simulink subsystem "Day2_Scenario_2_3"  (R2024a)
settings: Solver=VariableStepAuto  StartTime=0.0  StopTime=10.0  RelTol=1e-3
libraries: CarMaker4SL x5
settings Model: Creator=junhyung.cha  LastModifiedBy=User

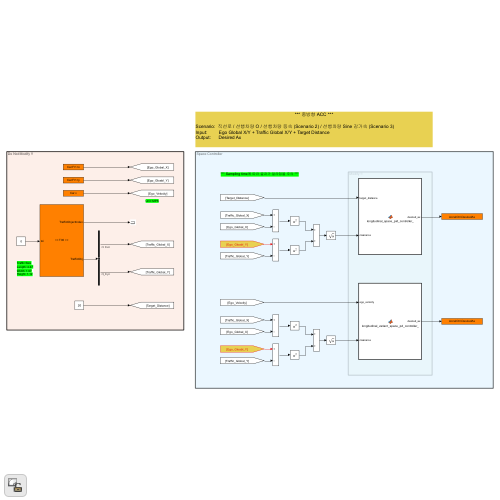
[thumbnail: Simulink's stored preview of the top-level diagram]
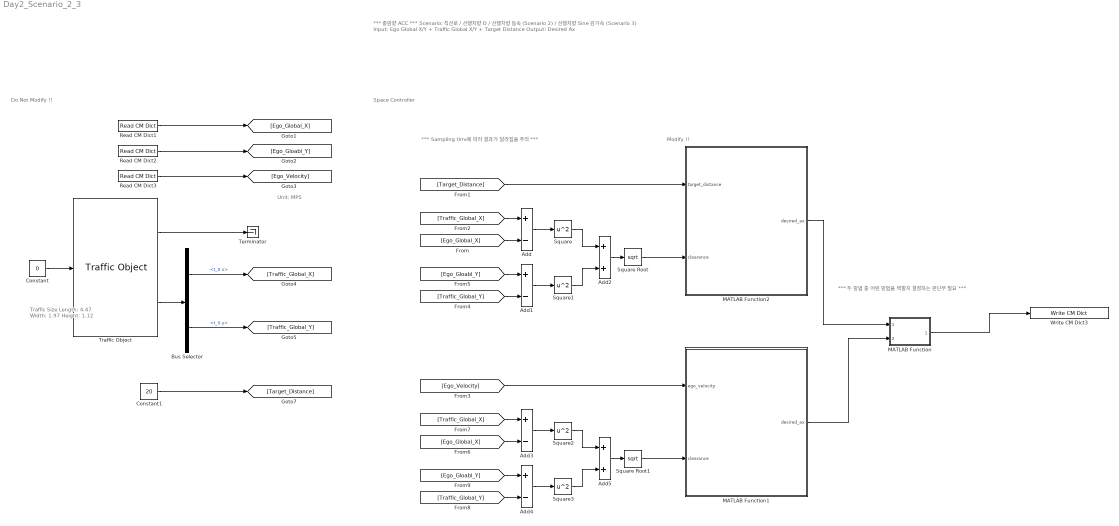
== system Day2_Scenario_2_3 ==
  note: *** Sampling time에 따라 결과가 달라짐을 주의 ***
  note: Space Controller
  note: Modify !!
  note: Do Not Modify !!
  note: Traffic Size
      | Length: 4.47
      | Width: 1.97
      | Height: 1.12
  note: *** 종방향 ACC ***
      |
      | Scenario: 직선로 / 선행차량 O / 선행차량 등속 (Scenario 2) / 선행차량 Sine 감가속 (Scenario 3)
      | Input: Ego Global X/Y + Traffic Global X/Y + Target Distance
      | Output: Desired Ax
  note: Unit: MPS
  note: *** 두 방법 중 어떤 방법을 택할지 결정하는 판단부 필요 ***
  Add{,1,3..4} (4 alike) : Sum  Inputs=+-
  Add2 : Sum
  Add5 : Sum
  Bus Selector : BusSelector  OutputSignals=t_0 x,t_0 y
  Constant : Constant  Value=0
  Constant1 : Constant  Value=20
  MATLAB Function : MATLAB Function  TreatAsAtomicUnit=on
  MATLAB Function1 : MATLAB Function  TreatAsAtomicUnit=on
  MATLAB Function2 : MATLAB Function  TreatAsAtomicUnit=on
  Read CM Dict1 : CarMaker4SL/Read CM Dict  xname=Car.Fr1.tx  xsync=off  xstime=Inherited
  Read CM Dict2 : CarMaker4SL/Read CM Dict  xname=Car.Fr1.ty  xsync=off  xstime=Inherited
  Read CM Dict3 : CarMaker4SL/Read CM Dict  xname=Car.v  xsync=off  xstime=Inherited
  Square{,1..3} (4 alike) : Math  Operator=square
  Square Root : Sqrt
  Square Root1 : Sqrt
  Terminator : Terminator
  Traffic Object : CarMaker4SL/Traffic Object  xname=T00  ximode=Traffic Id  xstime=Inherited
      settings: SourceProductName=CarMaker4SL
  Write CM Dict3 : CarMaker4SL/Write CM Dict  xname=AccelCtrl.DesiredAx  xsync=off
  wires:
  Read CM Dict2/1 -> [Ego_Gloabl_Y]
  Read CM Dict1/1 -> [Ego_Global_X]
  Constant/1 -> Traffic Object/1
  Traffic Object/2 -> Bus Selector/1
  Traffic Object/1 -> Terminator/1
  Bus Selector/1 -> [Traffic_Global_X]  "<t_0 x>"
  Bus Selector/2 -> [Traffic_Global_Y]  "<t_0 y>"
  Square Root/1 -> MATLAB Function2/2(clearance)
  Constant1/1 -> [Target_Distance]
  [Ego_Global_X] -> Add/2
  [Traffic_Global_X] -> Add/1
  [Traffic_Global_Y] -> Add1/2
  [Ego_Gloabl_Y] -> Add1/1
  Add1/1 -> Square1/1
  Add2/1 -> Square Root/1
  Square/1 -> Add2/1
  Square1/1 -> Add2/2
  [Target_Distance] -> MATLAB Function2/1(target_distance)
  Add/1 -> Square/1
  Read CM Dict3/1 -> [Ego_Velocity]
  [Ego_Velocity] -> MATLAB Function1/1(ego_velocity)
  Add3/1 -> Square2/1
  Square3/1 -> Add5/2
  Square2/1 -> Add5/1
  Add5/1 -> Square Root1/1
  Add4/1 -> Square3/1
  [Ego_Gloabl_Y] -> Add4/1
  [Traffic_Global_Y] -> Add4/2
  [Traffic_Global_X] -> Add3/1
  [Ego_Global_X] -> Add3/2
  Square Root1/1 -> MATLAB Function1/2(clearance)
  MATLAB Function/1(desired_ax) -> Write CM Dict3/1
  MATLAB Function1/1(desired_ax) -> MATLAB Function/2(desired_ax_2)
  MATLAB Function2/1(desired_ax) -> MATLAB Function/1(desired_ax_1)

== matlab function Day2_Scenario_2_3/MATLAB Function1 ==
  settings: updateMethod=DISCRETE  sampleTime=0.05
  data: ego_velocity input; desired_ax output; clearance input
function desired_ax = longitudinal_vant_space_pd_controller_(ego_velocity, clearance)

% Input
% ego_velocity : Ego vehicle speed [m/s]
% clearance    : 실제 차간거리 [m]
%
% Output
% desired_ax   : 요구 가속도 [m/s^2]

Ts = 0.01;   % Sampling time [s]

time_gap = 1.2;         % Time headway [s]
standstill_dist = 5.0;  % 정지 상태 최소 거리 [m]

Kp = 0.25;
Kd = 0.12;

ax_max = 1.5;
ax_min = -3.0;

persistent prev_error

% 속도 기반 목표 차간거리
target_distance = standstill_dist + time_gap * ego_velocity;

if isempty(prev_error)
    prev_error = clearance - target_distance;
end

% 거리 오차
% 양수: 실제 거리가 목표보다 큼 → 가속
% 음수: 실제 거리가 목표보다 작음 → 감속
error = clearance - target_distance;

% 오차 변화율
error_dot = (error - prev_error) / Ts;

% PD 제어
desired_ax = Kp * error + Kd * error_dot;

% 가속도 제한
if desired_ax > ax_max
    desired_ax = ax_max;
elseif desired_ax < ax_min
    desired_ax = ax_min;
end

prev_error = error;

end

== matlab function Day2_Scenario_2_3/MATLAB Function2 ==
  settings: updateMethod=DISCRETE  sampleTime=0.05
  data: target_distance input; desired_ax output; clearance input
function desired_ax = longitudinal_space_pid_controller_(target_distance, clearance)

% Input
% target_distance : 목표 차간거리 [m]
% clearance       : 실제 차간거리 [m]
%
% Output
% desired_ax      : 요구 가속도 [m/s^2]

Ts = 0.01;   % Sampling time [s], 모델 step time에 맞춰야 함

Kp = 0.25;
Ki = 0.02;
Kd = 0.10;

ax_max = 1.5;    % 최대 가속도
ax_min = -3.0;   % 최대 감속도

persistent prev_error error_sum

if isempty(prev_error)
    prev_error = clearance - target_distance;
    error_sum = 0;
end

% 거리 오차
% 양수: 앞차와 멂 → 가속 필요
% 음수: 앞차와 가까움 → 감속 필요
error = clearance - target_distance;

% 적분항
error_sum = error_sum + error * Ts;

% 적분항 과도 누적 방지
if error_sum > 50
    error_sum = 50;
elseif error_sum < -50
    error_sum = -50;
end

% 미분항
error_dot = (error - prev_error) / Ts;

% PID 제어
desired_ax = Kp * error + Ki * error_sum + Kd * error_dot;

% 가속도 제한
if desired_ax > ax_max
    desired_ax = ax_max;
elseif desired_ax < ax_min
    desired_ax = ax_min;
end

prev_error = error;

end

== matlab function Day2_Scenario_2_3/MATLAB Function ==
  data: desired_ax_1 input; desired_ax output; desired_ax_2 input
function desired_ax = acc_decision_(desired_ax_1, desired_ax_2)

% desired_ax_1 : 위쪽 거리 PID 제어기 출력
% desired_ax_2 : 아래쪽 속도기반 거리 PD 제어기 출력
% desired_ax   : 최종 AccelCtrl.DesiredAx 입력

% 두 제어기 중 더 보수적인 값 선택
desired_ax = min(desired_ax_1, desired_ax_2);

% 최종 가속도 제한
ax_max = 1.5;    % 최대 가속도 [m/s^2]
ax_min = -3.0;   % 최대 감속도 [m/s^2]

if desired_ax > ax_max
    desired_ax = ax_max;
elseif desired_ax < ax_min
    desired_ax = ax_min;
end

end
